simulink model "Lab1s"  (R2023b)
settings: Solver=VariableStepAuto  StartTime=0.0  StopTime=10.0  RelTol=1e-3
undefined symbols (not defined in the file): b, C_m, C_omega, J_dv, L_ov, L_ya, R_ya
settings Model: Creator=a2  LastModifiedBy=a2

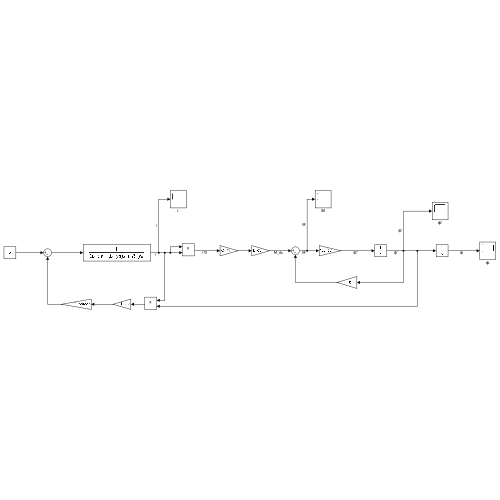
[thumbnail: Simulink's stored preview of the top-level diagram]
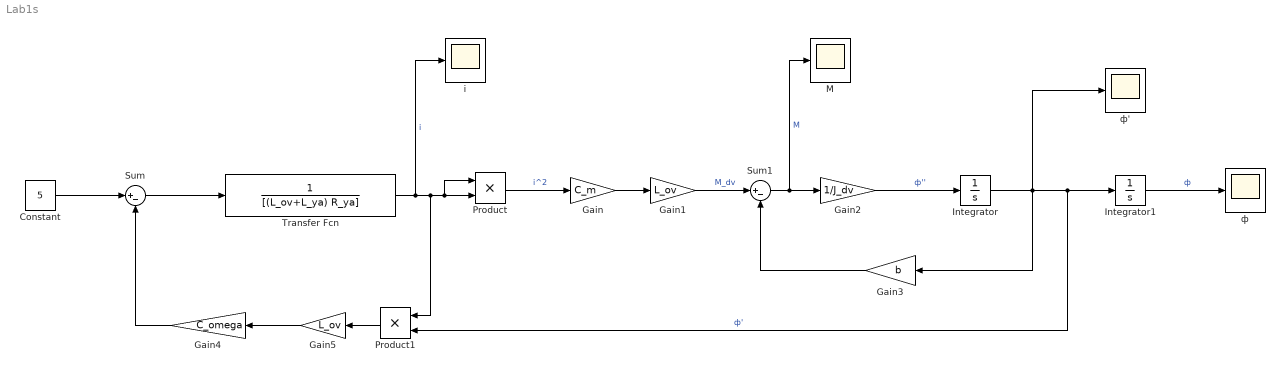
== system Lab1s ==
  Constant : Constant  Value=5
  Gain : Gain  Gain=C_m
  Gain1 : Gain  Gain=L_ov
  Gain2 : Gain  Gain=1/J_dv
  Gain3 : Gain  Gain=b
  Gain4 : Gain  Gain=C_omega
  Gain5 : Gain  Gain=L_ov
  Integrator : Integrator
  Integrator1 : Integrator
  M : Scope
  Product : Product
  Product1 : Product
  Sum : Sum  Inputs=|+-
  Sum1 : Sum  Inputs=|+-
  Transfer Fcn : TransferFcn  Denominator=[(L_ov+L_ya) R_ya]
  i : Scope
  ф : Scope
  ф' : Scope
  wires:
  Constant/1 -> Sum/1
  Sum/1 -> Transfer Fcn/1
  Transfer Fcn/1 -> i/1, Product1/1, Product/1, Product/2  "i"
  Product/1 -> Gain/1  "i^2"
  Gain/1 -> Gain1/1
  Gain2/1 -> Integrator/1  "ф''"
  Integrator/1 -> Gain3/1, ф'/1, Product1/2, Integrator1/1  "ф'"
  Integrator1/1 -> ф/1  "ф"
  Gain5/1 -> Gain4/1
  Product1/1 -> Gain5/1
  Gain4/1 -> Sum/2
  Sum1/1 -> M/1, Gain2/1  "M"
  Gain1/1 -> Sum1/1  "M_dv"
  Gain3/1 -> Sum1/2
